simulink model "Schleudersitz_2310"  (R2021a)
settings: Solver=VariableStepAuto  StartTime=0.0  StopTime=300  RelTol=1e-3
libraries: simulink x10
settings Model: SimulationMode=accelerator  Creator=tobia  LastModifiedBy=tobia
settings SolverCC: AlgebraicLoopSolver=TrustRegion
settings DebuggingCC: SFMachineParentedDataDiag=warning

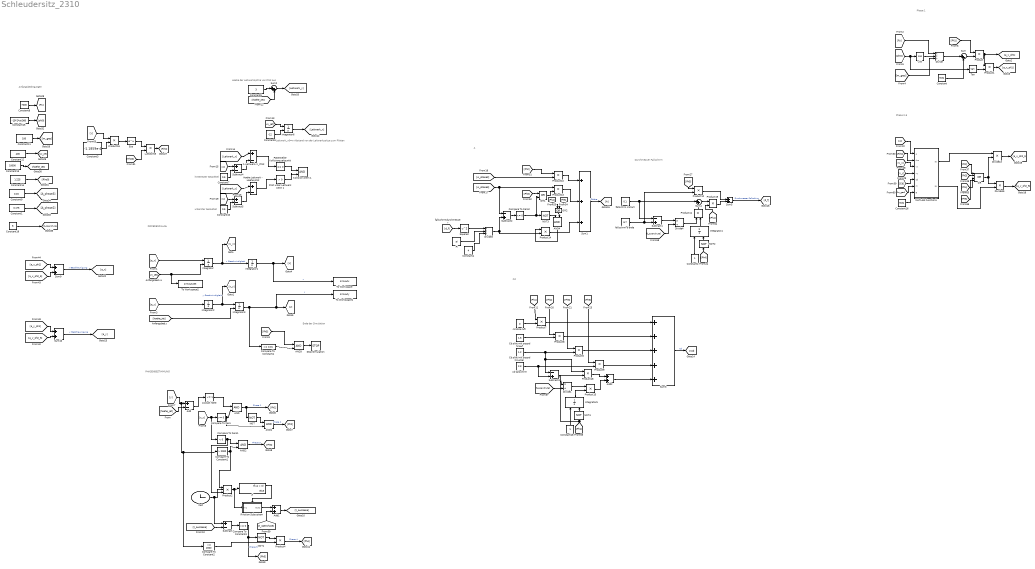
== system Schleudersitz_2310 ==
  note: Hoehe der Leitwerkspitze von Pilot aus
  note: unterster Sesselteil
  note: Leitwerk_x0=x-Abstand von der Leitwerkspitze zum Piloten
  note: Durchmesser Fallschirm
  note: A
  note: Cd
  note: Ende der Simulation
  note: DIFFERENZIALGL
  note: PHASENBESTIMMUNG
  note: Phase 2-5
  note: Anfangsbedingungen
  note: Phase 1
  note: hinterester Sesselteil
  AND{,1..4} (5 alike) : Logic  IconShape=distinctive  AllPortsSameDT=off  OutDataTypeStr=boolean
  Add : Sum  Inputs=+-
  Add1 : Sum
  Add2 : Sum
  Cd pilot mit sessel hinauf : Constant  Value=1.6
  Cd pilot mit sessel hinunter : Constant  Value=1.2
  Compare To Constant1 : simulink/Logic and Bit Operations/Compare To Constant  relop=>  const=2000  OutDataTypeStr=boolean
  Compare To Constant2 : simulink/Logic and Bit Operations/Compare To Constant  relop=<=  const=2000  OutDataTypeStr=boolean
  Compare To Constant3 : simulink/Logic and Bit Operations/Compare To Constant  relop=>=  const=0  OutDataTypeStr=boolean
  Compare To Constant4 : simulink/Logic and Bit Operations/Compare To Constant  relop=<=  const=0.01  OutDataTypeStr=boolean
  Compare To Zero : simulink/Logic and Bit Operations/Compare To Zero  relop=>=  OutDataTypeStr=boolean
  Compare To Zero1 : simulink/Logic and Bit Operations/Compare To Zero  relop=<  OutDataTypeStr=boolean
  Compare To Zero2 : simulink/Logic and Bit Operations/Compare To Zero  relop=<=  OutDataTypeStr=boolean
  Constant : Constant  Value=9.81
  Constant1 : Constant  Value=0.175
  Constant10 : Constant  Value=0.5
  Constant11 : Constant  Value=100
  Constant12 : Constant  Value=400
  Constant13 : Constant  Value=10000
  Constant14 : Constant  Value=1.225
  Constant15 : Constant  Value=-15*2*pi/360
  Constant16 : Constant  Value=9.81
  Constant18 : Constant
  Constant19 : Constant  Value=6
  Constant2 : Constant
  Constant3 : Constant  Value=-1.1859e-4
  Constant4 : Constant  Value=4
  Constant5 : Constant  Value=3
  Constant6 : Constant  Value=-12
  Constant7 : Constant  Value=0.5
  Constant8 : Constant  Value=7000
  Constant9 : Constant  Value=0.15
  Cos : Trigonometry  Operator=cos
  Divide : Product  Inputs=**/
  Divide1 : Product  Inputs=*/
  Divide13 : Product  Inputs=**
  Divide15 : Product  Inputs=**
  Divide3 : Product  Inputs=**/
  Divide4 : Product  Inputs=*/
  Exp : Math  SaturateOnIntegerOverflow=on
  Hoehe Leitwerk - Hoehe pilot : Sum  Inputs=|+-
  If : If
  If Action Subsystem : Subsystem  TreatAsAtomicUnit=on
  Integrator : Integrator  InitialConditionSource=external
  Integrator1 : Integrator
  Integrator2 : Integrator
  Integrator3 : Integrator  InitialConditionSource=external
  Integrator4 : Integrator  ExternalReset=level
  Integrator5 : Integrator  ExternalReset=level
  Integrator6 : Integrator  InitialConditionSource=external
  Kollision wenn 1 : Logic  IconShape=distinctive  AllPortsSameDT=off  OutDataTypeStr=boolean
  Luftdichte : Product
  MATLAB Function1 : MATLAB Function  TreatAsAtomicUnit=on
  NOT{,1..4} (5 alike) : Logic  Operator=NOT  IconShape=distinctive  AllPortsSameDT=off  OutDataTypeStr=boolean
  OR : Logic  Operator=OR  Inputs=4  IconShape=distinctive  AllPortsSameDT=off  OutDataTypeStr=boolean
  OR1 : Logic  Operator=OR  IconShape=distinctive  AllPortsSameDT=off  OutDataTypeStr=boolean
  OR2 : Logic  Operator=OR  IconShape=distinctive  AllPortsSameDT=off  OutDataTypeStr=boolean
  Pi : Constant  Value=pi  OutDataTypeStr=Inherit: Inherit via back propagation
  Pilot unter Leitwerk wenn 1 : simulink/Logic and Bit Operations/Compare To Zero  relop=>  OutDataTypeStr=boolean
  Potentieller Kollisionszeitpunkt : simulink/Logic and Bit Operations/Compare To Zero  relop===  OutDataTypeStr=boolean
  Product{,1,4,6..16,18..19} (16 alike) : Product
  Product2 : Product  Inputs=3
  Square2 : Math  Operator=square  SaturateOnIntegerOverflow=on
  Stop Simulation : Stop
  Subtract : Sum  Inputs=+-
  Subtract1 : Sum  Inputs=-+
  Subtract2 : Sum  Inputs=-+
  Subtract3 : Sum  Inputs=-+
  Subtract4 : Sum  Inputs=+-
  Subtract5 : Sum  Inputs=+-
  Sum : Sum  Inputs=|+-
  Sum1 : Sum  Inputs=+++
  Sum10 : Sum
  Sum2 : Sum  Inputs=|++
  Sum3 : Sum  Inputs=+++++
  Sum4 : Sum  Inputs=|++
  Sum5 : Sum
  Sum9 : Sum
  Tan : Trigonometry  Operator=tan
  To Workspace : ToWorkspace  VariableName=simoutx  SaveFormat=Structure With Time  SampleTime=-1
  To Workspace1 : ToWorkspace  VariableName=simouty  SaveFormat=Structure With Time  SampleTime=-1
  To Workspace2 : ToWorkspace  VariableName=simoutvjet  SaveFormat=Structure With Time  SampleTime=-1
  X-Leitwerk-X_Pilot : Sum  Inputs=|+-
  Zeit : Clock
  cd fallschirm : Constant  Value=2.3
  cd ohne luft : Constant  Value=0
  cockpit höhe : simulink/Logic and Bit Operations/Compare To Constant  relop=<=  const=1  OutDataTypeStr=boolean
  fallschrm d ende : Constant  Value=6.7
  fallschrm d start : Constant  Value=0.1
  wires:
  [a_x] -> Integrator/1
  Integrator/1 -> [v_x], Integrator1/1  "x Geschwindigkeit"
  [a_y] -> Integrator2/1
  Integrator2/1 -> [v_y], Integrator3/1  "y Geschwindigkeit"
  Constant/1 -> Sum/2
  [Fs] -> Divide/1
  [phi0] -> Tan/1, Cos/1
  Cos/1 -> Divide/2
  [m_ges] -> Divide/3
  Divide/1 -> Sum/1
  [Ph1] -> Product/1
  Sum/1 -> Product/2
  Product/1 -> Product1/1, [a_y_ph1]
  Tan/1 -> Product1/2
  Integrator1/1 -> To Workspace/1, [x]  "x"
  [y] -> Compare To Constant2/1, Compare To Constant1/1, Add/1
  [hoehe_jet] -> Add/2
  Add/1 -> cockpit höhe/1
  [v_y] -> Compare To Zero1/1, Compare To Zero/1
  Compare To Zero/1 -> AND/2, AND1/2
  cockpit höhe/1 -> AND/1
  AND/1 -> NOT/1, [Ph1]  "Phase 1"
  NOT/1 -> AND1/1
  AND1/1 -> [Ph2]  "Phase 2"
  Compare To Zero1/1 -> Product2/3, AND2/1
  Compare To Constant1/1 -> Product2/1, AND2/2
  AND2/1 -> [Ph3]  "Phase 3"
  Zeit/1 -> Subtract/1, Product2/2
  Product2/1 -> If Action Subsystem/1(In1), If/1
  If/1 -> If Action Subsystem/Action
  If Action Subsystem/1(Out1) -> Add1/1
  [t_openchute] -> Add1/2
  Add1/1 -> [t_ausloese]
  [t_ausloese] -> Subtract/2
  Subtract/1 -> Compare To Constant3/1
  Compare To Constant3/1 -> [Ph5], NOT1/1  "Phase 5"
  Compare To Constant2/1 -> Product4/2
  NOT1/1 -> Product4/1
  Product4/1 -> [Ph4]  "Phase 4"
  Compare To Constant4/1 -> AND3/2
  Integrator3/1 -> Compare To Constant4/1, To Workspace1/1, [y]  "y"
  [Ph5] -> AND3/1
  AND3/1 -> Stop Simulation/1
  Product1/1 -> [a_x_ph1]
  [vx_jet] -> To Workspace2/1, Integrator/2
  [hoehe_jet] -> Integrator3/2
  Cd pilot mit sessel hinunter/1 -> Product6/2, Product18/1, Subtract3/1
  cd ohne luft/1 -> Product7/2
  [Ph1] -> Product7/1
  Product7/1 -> Sum3/1
  [Ph2] -> Product8/1
  Cd pilot mit sessel hinauf/1 -> Product8/2
  Product8/1 -> Sum3/2
  [Ph3] -> Product6/1
  Product6/1 -> Sum3/3
  cd fallschirm/1 -> Product9/2, Subtract3/2
  [Ph5] -> Product9/1
  Product9/1 -> Sum3/4
  Sum3/1 -> [Cd]  "Cd"
  [d_f] -> Square2/1
  Square2/1 -> Divide3/1
  Constant4/1 -> Divide3/3
  Pi/1 -> Divide3/2
  Divide3/1 -> Product14/2, Subtract2/2
  fallschrm d start/1 -> Subtract1/1, Sum4/1
  fallschrm d ende/1 -> Product12/2, Subtract1/2
  [t_openchute] -> Divide4/2
  Subtract1/1 -> Divide4/1
  Divide4/1 -> Product11/1
  Product11/1 -> Sum4/2
  Constant2/1 -> Integrator4/1
  [Ph4] -> NOT2/1
  NOT2/1 -> Integrator4/2
  Integrator4/1 -> Product11/2
  [Ph5] -> Product12/1
  Product12/1 -> Sum5/1
  Sum5/1 -> [d_f]  "Durchmesser Fallschirm"
  [Cd] -> MATLAB Function1/5(cd)
  [A] -> MATLAB Function1/1(A)
  [v_y] -> MATLAB Function1/4(vy)
  [Rho] -> MATLAB Function1/2(rho)
  [v_x] -> MATLAB Function1/3(vx)
  [a_x_ph2_5] -> Sum9/2
  [a_x_ph1] -> Sum9/1
  Sum9/1 -> [a_x]  "x Beschleunigung"
  Sum10/1 -> [a_y]  "y Beschleunigung"
  [a_y_ph1] -> Sum10/1
  Constant8/1 -> [Fs]
  Constant11/1 -> [m_ges]
  Constant12/1 -> [vx_jet]
  Constant13/1 -> [hoehe_jet]
  Constant14/1 -> [Rho0]
  Constant15/1 -> [phi0]
  Constant16/1 -> MATLAB Function1/7(g)
  [m_ges] -> MATLAB Function1/6(m)
  Divide13/1 -> [a_x_ph2_5]
  MATLAB Function1/2(ay) -> Divide15/2
  Divide15/1 -> [a_y_ph2_5]
  [Ph2] -> Product10/1
  [A_phase2] -> Product10/2
  [Ph3] -> OR1/1
  [A_phase3] -> Subtract2/1, Product13/1
  OR1/1 -> Product13/2
  Subtract2/1 -> Compare To Zero2/1
  Compare To Zero2/1 -> OR1/2, NOT3/1
  NOT3/1 -> AND4/1
  Product14/1 -> Sum1/3
  Product10/1 -> Sum1/1
  Product13/1 -> Sum1/2
  Sum1/1 -> [A]  "Fläche"
  [Ph4] -> OR2/1
  AND4/1 -> Product14/1
  [Ph5] -> OR2/2
  OR2/1 -> AND4/2
  Constant1/1 -> [A_phase2]
  Constant9/1 -> [A_phase3]
  NOT4/1 -> Integrator5/2
  Constant18/1 -> Integrator5/1
  Subtract3/1 -> Divide1/1
  [t_openchute] -> Divide1/2
  Constant19/1 -> [t_openchute]
  Divide1/1 -> Product15/1
  Integrator5/1 -> Product15/2
  Product15/1 -> Add2/2
  Add2/1 -> Sum3/5
  Constant3/1 -> Product16/2
  [y] -> Product16/1
  Product16/1 -> Exp/1
  Exp/1 -> Luftdichte/1
  [Rho0] -> Luftdichte/2
  Luftdichte/1 -> [Rho]
  Product18/1 -> Add2/1
  [Ph4] -> NOT4/1, Product18/2
  Sum4/1 -> Product19/1
  Product19/1 -> Sum5/2
  [Ph4] -> Product19/2
  [Ph2] -> OR/1
  [Ph3] -> OR/2
  [Ph4] -> OR/3
  [Ph5] -> OR/4
  OR/1 -> Divide13/2, Divide15/1
  MATLAB Function1/1(ax) -> Divide13/1
  [a_y_ph2_5] -> Sum10/2
  Constant5/1 -> Sum2/1
  [hoehe_jet] -> Sum2/2
  Sum2/1 -> [Leitwerk_y]
  Constant6/1 -> Integrator6/2
  [vx_jet] -> Integrator6/1
  Integrator6/1 -> [Leitwerk_x]
  X-Leitwerk-X_Pilot/1 -> Potentieller Kollisionszeitpunkt/1
  [Leitwerk_x] -> X-Leitwerk-X_Pilot/1
  Potentieller Kollisionszeitpunkt/1 -> Kollision wenn 1/1
  [Leitwerk_y] -> Hoehe Leitwerk - Hoehe pilot/1
  Hoehe Leitwerk - Hoehe pilot/1 -> Pilot unter Leitwerk wenn 1/1
  Pilot unter Leitwerk wenn 1/1 -> Kollision wenn 1/2
  [x] -> Subtract4/1
  Constant7/1 -> Subtract4/2
  Subtract4/1 -> X-Leitwerk-X_Pilot/2
  Subtract5/1 -> Hoehe Leitwerk - Hoehe pilot/2
  Constant10/1 -> Subtract5/2
  [y] -> Subtract5/1

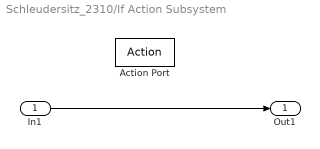
== system Schleudersitz_2310/If Action Subsystem ==
  In1 : Inport
  Action Port : ActionPort  ActionPortLabel=if(u1 > 0)
  Out1 : Outport
  wires:
  In1/1 -> Out1/1

== matlab function Schleudersitz_2310/MATLAB Function1 ==
  data: A input; ax output; rho input; vx input; vy input; cd input; m input; g input; ay output
function [ax,ay] = fcn(A,rho,vx,vy,cd,m,g)
coder.extrinsic('solveSym_Ph2');
ax=0;
ay=0;
[ax,ay]= solveSym_Ph2(A,rho,vx,vy,cd,m,g);
end
